simulink model "PIDsimu"  (R2016a)
settings: Solver=ode45  StartTime=0.0  StopTime=030  RelTol=1e-3
values from neighbouring files (symbols this model uses):
  A = double(subs(jacobian(F_EOM_Nonlin, states), [states, ctrl_input, design_para], [0, theta_e, 0, 0, 0, 0,F_1_e,F_2_e,beta_1_e,beta_2_e,design_var]))    [Copy_of_EOM.m]    (also in EOM.m = double(subs(jacobian(F_EOM_Nonlin, states), [states, ctrl_in; PID_Tuning.m; wingarea.m = 0.5232)
  B = double(subs(jacobian(F_EOM_Nonlin, ctrl_input), [states, ctrl_input, design_para], [0, theta_e, 0, 0, 0, 0,F_1_e,F_2_e,beta_1_e,beta_2_e,design_var]))    [Copy_of_EOM.m]    (also in EOM.m = double(subs(jacobian(F_EOM_Nonlin, ctrl_input), [states, ctr; PID_Tuning.m)
  C = eye(6)    [Copy_of_EOM.m]    (also in EOM.m; PID_Tuning.m)
  D = zeros(6,4)    [Copy_of_EOM.m]    (also in EOM.m; PID_Tuning.m)
libraries: simulink x5
settings Model: Creator=zhang794  LastModifiedBy=AutoLab Mous 3
settings DataIOCC: LimitDataPoints=on  SaveFormat=Array
settings DebuggingCC: AllowSymbolicDim=off
settings HardwareCC: ProdBitPerPointer=32  ProdLargestAtomicFloat=None  ProdIntDivRoundTo=Undefined  ProdEndianess=Unspecified  ProdWordSize=32  ProdHWDeviceType=32-bit Generic
settings ModelReferenceCC: PropagateSignalLabelsOutOfModel=off
settings ConfigComp: CovModelRefEnable=Off

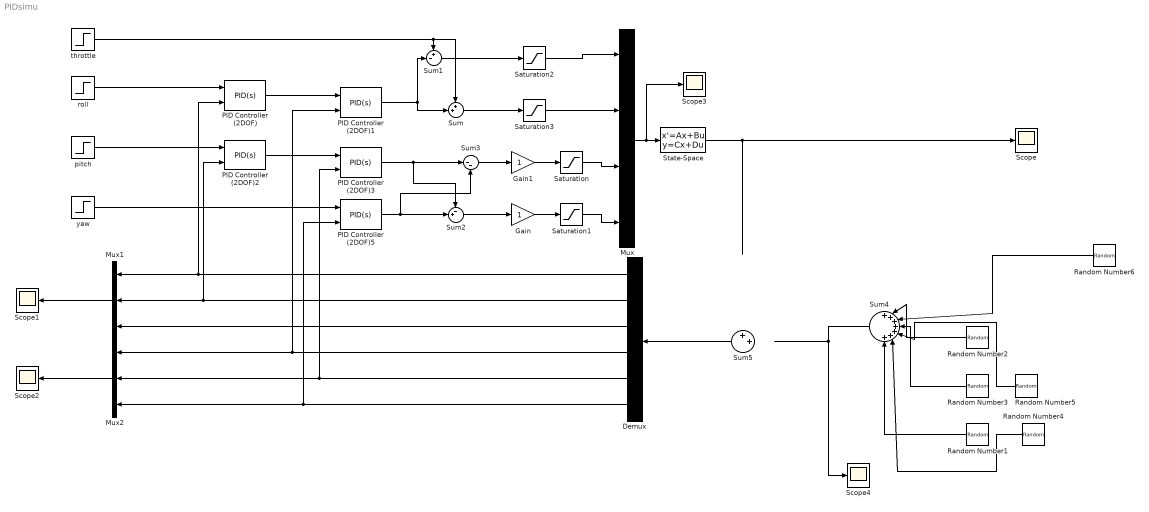
== system PIDsimu ==
  Demux : Demux  Outputs=6
  Gain : Gain
  Gain1 : Gain
  Mux : Mux
  Mux1 : Mux  Inputs=3
  Mux2 : Mux  Inputs=3
  PID Controller (2DOF){,1..3,5} (5 alike) : simulink/Continuous/PID Controller (2DOF)  Controller=PID  TimeDomain=Continuous-time  SampleTime=-1  IntegratorMethod=Forward Euler  FilterMethod=Forward Euler  Form=Parallel  UseFilter=on  ControllerParametersSource=internal  P=0.7  I=0  D=0  N=1  b=1  c=1  InitialConditionSource=internal  InitialConditionForIntegrator=0  InitialConditionForFilter=0  ExternalReset=none  LimitOutput=off  UpperSaturationLimit=inf  LowerSaturationLimit=-inf  LinearizeAsGain=on  AntiWindupMode=none  Kb=1  TrackingMode=off  Kt=1  PParamMin=[]  PParamMax=[]  IParamMin=[]  IParamMax=[]  DParamMin=[]  DParamMax=[]  NParamMin=[]  NParamMax=[]  bParamMin=[]  bParamMax=[]  cParamMin=[]  cParamMax=[]  KbParamMin=[]  KbParamMax=[]  KtParamMin=[]  KtParamMax=[]  POutMin=[]  POutMax=[]  IOutMin=[]  IOutMax=[]  DOutMin=[]  DOutMax=[]  NOutMin=[]  NOutMax=[]  bOutMin=[]  bOutMax=[]  cOutMin=[]  cOutMax=[]  KbOutMin=[]  KbOutMax=[]  KtOutMin=[]  KtOutMax=[]  IntegratorOutMin=[]  IntegratorOutMax=[]  FilterOutMin=[]  FilterOutMax=[]  SumOutMin=[]  SumOutMax=[]  Sum1OutMin=[]  Sum1OutMax=[]  Sum2OutMin=[]  Sum2OutMax=[]  Sum3OutMin=[]  Sum3OutMax=[]  SumI1OutMin=[]  SumI1OutMax=[]  SumI2OutMin=[]  SumI2OutMax=[]  SumI3OutMin=[]  SumI3OutMax=[]  SumDOutMin=[]  SumDOutMax=[]  SaturationOutMin=[]  SaturationOutMax=[]  IntegratorContinuousStateAttributes=''  IntegratorStateMustResolveToSignalObject=off  IntegratorRTWStateStorageClass=Auto  FilterContinuousStateAttributes=''  FilterStateMustResolveToSignalObject=off  FilterRTWStateStorageClass=Auto  DifferentiatorICPrevScaledInput=0  DifferentiatorOutMin=[]  DifferentiatorOutMax=[]
  Random Number1 : RandomNumber  Mean=[0;0;0;0;0;0.]  Variance=[0 0 0.0001 0 0 0]  Seed=1363  SampleTime=0
  Random Number2 : RandomNumber  Mean=[0;0;0;0;0;0.]  Variance=[0.0001 0 0 0 0 0]  Seed=2535  SampleTime=0
  Random Number3 : RandomNumber  Mean=[0;0;0;0;0;0.]  Variance=[0 0.0001 0 0 0 0]  Seed=5747  SampleTime=0
  Random Number4 : RandomNumber  Mean=[0;0;0;0;0;0.]  Variance=[0 0 0 0.0033/4 0 0]  Seed=136613  SampleTime=0
  Random Number5 : RandomNumber  Mean=[0;0;0;0;0;0.]  Variance=[0 0 0 0 0.0033/4 0]  Seed=3535  SampleTime=0
  Random Number6 : RandomNumber  Mean=[0;0;0;0;0;0.]  Variance=[0 0 0 0 0 0.0033/4]  Seed=436346  SampleTime=0
  Saturation : Saturate
  Saturation1 : Saturate
  Saturation2 : Saturate  UpperLimit=15  LowerLimit=0
  Saturation3 : Saturate  UpperLimit=15  LowerLimit=0
  Scope{,1..4} (5 alike) : Scope
  State-Space : StateSpace  A=A  B=B  C=C  D=D  X0=[0.2 0.3 0 0 0 0]
  Sum : Sum  Inputs=++|
  Sum1 : Sum  Inputs=+-|
  Sum2 : Sum  Inputs=-+|
  Sum3 : Sum  Inputs=|--
  Sum4 : Sum  Inputs=+++++++
  Sum5 : Sum  Inputs=++|
  pitch : Step  Time=0  After=0  SampleTime=0
  roll : Step  Before=0.0  After=0.2  SampleTime=0
  throttle : Step  Time=0  After=10  SampleTime=0
  yaw : Step  Before=1  After=0  SampleTime=0
  wires:
  roll/1 -> PID Controller (2DOF)/1
  PID Controller (2DOF)/1 -> PID Controller (2DOF)1/1
  PID Controller (2DOF)1/1 -> Sum1/2, Sum/2
  PID Controller (2DOF)2/1 -> PID Controller (2DOF)3/1
  yaw/1 -> PID Controller (2DOF)5/1
  Sum/1 -> Saturation3/1
  Sum1/1 -> Saturation2/1
  PID Controller (2DOF)3/1 -> Sum2/1, Sum3/1
  PID Controller (2DOF)5/1 -> Sum3/2, Sum2/2
  Sum2/1 -> Gain/1
  Mux/1 -> Scope3/1, State-Space/1
  State-Space/1 -> Scope/1
  pitch/1 -> PID Controller (2DOF)2/1
  Gain/1 -> Saturation1/1
  Sum3/1 -> Gain1/1
  Gain1/1 -> Saturation/1
  Demux/1 -> PID Controller (2DOF)/2, Mux1/1
  Demux/2 -> PID Controller (2DOF)2/2, Mux1/2
  Demux/4 -> Mux2/1, PID Controller (2DOF)1/2
  Demux/5 -> Mux2/2, PID Controller (2DOF)3/2
  Demux/6 -> Mux2/3, PID Controller (2DOF)5/2
  throttle/1 -> Sum1/1, Sum/1
  Demux/3 -> Mux1/3
  Sum4/1 -> Scope4/1
  Random Number2/1 -> Sum4/2
  Random Number6/1 -> Sum4/3
  Random Number3/1 -> Sum4/4
  Random Number5/1 -> Sum4/5
  Random Number4/1 -> Sum4/6
  Random Number1/1 -> Sum4/7
  Mux2/1 -> Scope2/1
  Mux1/1 -> Scope1/1
  Saturation1/1 -> Mux/4
  Saturation/1 -> Mux/3
  Saturation3/1 -> Mux/2
  Saturation2/1 -> Mux/1
  Sum5/1 -> Demux/1
